simulink model "XorGateNand"  (R2024b)
settings: Solver=VariableStepAuto  StartTime=0.0  StopTime=inf  RelTol=1e-3

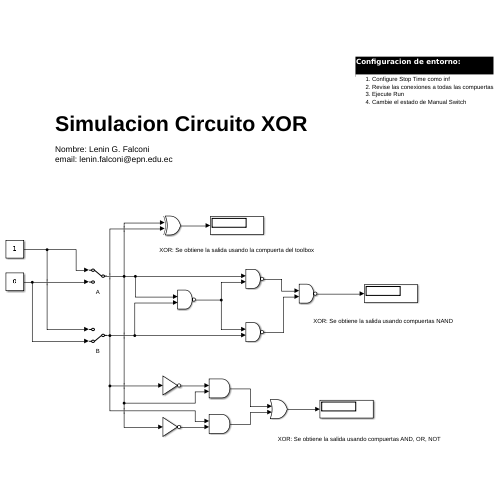
[thumbnail: Simulink's stored preview of the top-level diagram]
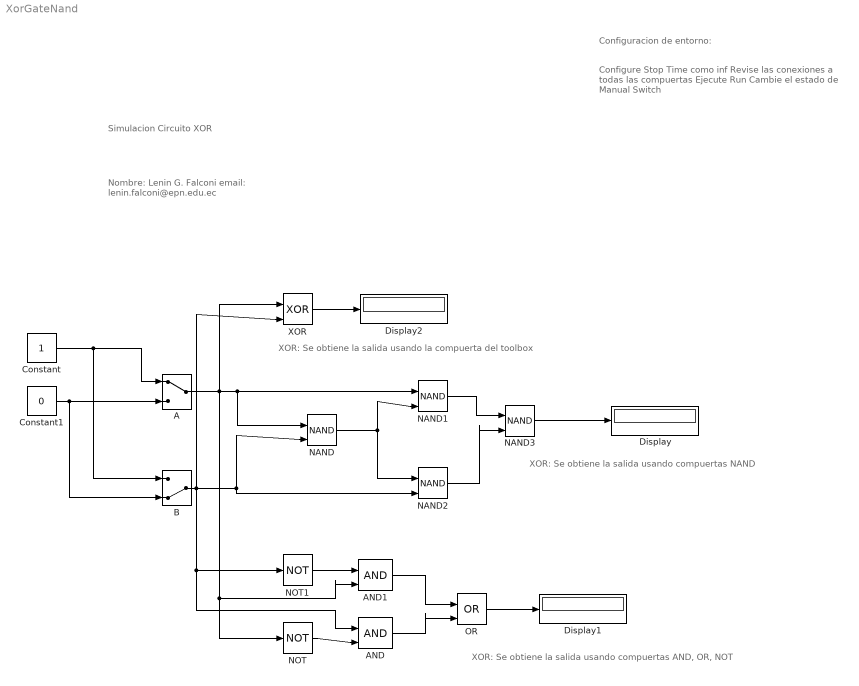
== system XorGateNand ==
  note: Configure Stop Time como inf
      | Revise las conexiones a todas las compuertas
      | Ejecute Run
      | Cambie el estado de Manual Switch
  note: Configuracion de entorno:
  note: Nombre: Lenin G. Falconi
      | email: lenin.falconi@epn.edu.ec
  note: Simulacion Circuito XOR
  note: XOR: Se obtiene la salida usando la compuerta del toolbox
  note: XOR: Se obtiene la salida usando compuertas NAND
  note: XOR: Se obtiene la salida usando compuertas AND, OR, NOT
  A : ManualSwitch
  AND : Logic  IconShape=distinctive  AllPortsSameDT=off  OutDataTypeStr=boolean
  AND1 : Logic  IconShape=distinctive  AllPortsSameDT=off  OutDataTypeStr=boolean
  B : ManualSwitch  CurrentSetting=0
  Constant : Constant
  Constant1 : Constant  Value=0
  Display : Display
  Display1 : Display
  Display2 : Display
  NAND{,1..3} (4 alike) : Logic  Operator=NAND  IconShape=distinctive  AllPortsSameDT=off  OutDataTypeStr=boolean
  NOT : Logic  Operator=NOT  IconShape=distinctive  AllPortsSameDT=off  OutDataTypeStr=boolean
  NOT1 : Logic  Operator=NOT  IconShape=distinctive  AllPortsSameDT=off  OutDataTypeStr=boolean
  OR : Logic  Operator=OR  IconShape=distinctive  AllPortsSameDT=off  OutDataTypeStr=boolean
  XOR : Logic  Operator=XOR  IconShape=distinctive  AllPortsSameDT=off  OutDataTypeStr=boolean
  wires:
  NAND1/1 -> NAND3/1
  NAND2/1 -> NAND3/2
  NAND/1 -> NAND2/1, NAND1/2
  NAND3/1 -> Display/1
  Constant/1 -> B/1, A/1
  A/1 -> XOR/1, NOT/1, AND1/2, NAND/1, NAND1/1
  B/1 -> XOR/2, AND/1, NOT1/1, NAND2/2, NAND/2
  Constant1/1 -> B/2, A/2
  NOT/1 -> AND/2
  NOT1/1 -> AND1/1
  AND1/1 -> OR/1
  AND/1 -> OR/2
  OR/1 -> Display1/1
  XOR/1 -> Display2/1
